simulink model "GalvoModel_v60"  (R2015a)
settings: Solver=ode45  StartTime=0.0  StopTime=5  MaxStep=1e-4  RelTol=1e-3
InitFcn:
  | param=evalin('base','param;');
  | 
  | JR=str2num(param.JR);
  | KMT=str2num(param.KMT);
  | Rc=str2num(param.Rc);
  | Lc=str2num(param.Lc);
  | KFR=str2num(param.KFR);
  | KTB=str2num(param.KTB);
  | KBM=str2num(param.KBM);
  | Rsh=str2num(param.Rsh);
StartFcn:
  | sprintf('Info (%s):\nKTB = %.1e\nKBM = %.1e\n', gcs, KTB, KBM)
model workspace (MATLAB code in the model file):
  | %param=evalin('base','loadGalvoParam(4);');
  | param=evalin('base','param;');
  | 
  | JR=str2num(param.JR);
  | KMT=str2num(param.KMT);
  | Rc=str2num(param.Rc);
  | Lc=str2num(param.Lc);
  | KFR=str2num(param.KFR);
  | KTB=str2num(param.KTB);
  | KBM=str2num(param.KBM);
  | Rsh=str2num(param.Rsh);
undefined symbols (not defined in the file): FS
settings Model: Creator=mainster  LastModifiedBy=mainster
settings DataIOCC: SaveOutput=off  SaveTime=off
settings OptimizationCC: InlineParams=on  BufferReuse=off
settings DebuggingCC: UnderspecifiedInitializationDetection=Classic  MergeDetectMultiDrivingBlocksExec=none  SolverPrmCheckMsg=warning  StateNameClashWarn=warning  InitInArrayFormatMsg=none
settings ModelReferenceCC: ModelReferenceMinAlgLoopOccurrences=on

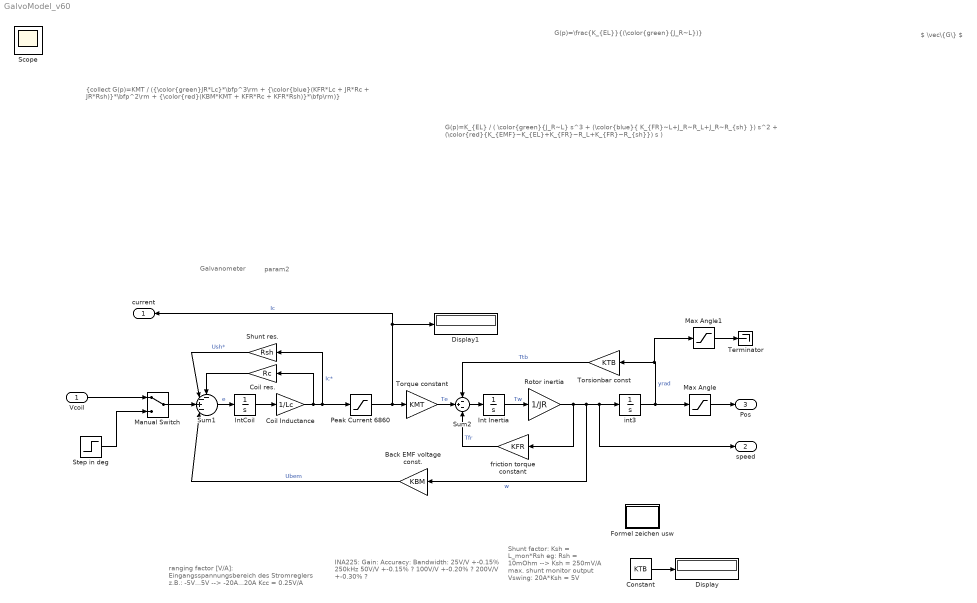
== system GalvoModel_v60 ==
  note: $ \vec\{G\} $
  note: G(p)=\frac{K_{EL}}{(\color{green}{J_R~L})}
  note: G(p)=K_{EL} / ( \color{green}{J_R~L} s^3 + (\color{blue}{ K_{FR}~L+J_R~R_L+J_R~R_{sh} }) s^2 + (\color{red}{K_{EMF}~K_{EL}+K_{FR}~R_L+K_{FR}~R_{sh}}) s )
  note: {collect G(p)=KMT / ({\color{green}JR*Lc}*\bfp^3\rm + {\color{blue}(KFR*Lc + JR*Rc + JR*Rsh)}*\bfp^2\rm + {\color{red}(KBM*KMT + KFR*Rc + KFR*Rsh)}*\bfp\rm)}
  note: param2
  note: Galvanometer
  note: ranging factor [V/A]:
      | Eingangsspannungsbereich des
      | Stromreglers z.B.:
      | -5V...5V --> -20A...20A
      | Kcc = 0.25V/A
  note: Shunt factor:
      | Ksh = L_mon*Rsh
      |
      | eg: Rsh = 10mOhm
      |
      | --> Ksh = 250mV/A
      | max. shunt monitor
      | output Vswing:
      | 20A*Ksh = 5V
  note: INA225:
      | Gain:		Accuracy:		Bandwidth:
      | 25V/V		+-0.15%		250kHz
      | 50V/V		+-0.15%		?
      | 100V/V	+-0.20%		?
      | 200V/V	+-0.30%		?
  Vcoil : Inport
  Back EMF voltage const. : Gain  Gain=KBM
  Coil Inductance : Gain  Gain=1/Lc
  Coil res. : Gain  Gain=Rc
  Constant : Constant  Value=KTB  SampleTime=-1
  Display : Display
  Display1 : Display
  Formel zeichen usw : Subsystem
  Int Inertia : Integrator
  IntCoil : Integrator
  Manual Switch : ManualSwitch
  Max Angle : Saturate  UpperLimit=20*pi/180  LowerLimit=-20*pi/180
      settings: AttributesFormatString=Max=%<UpperLimit>\nMin=%<LowerLimit>
  Max Angle1 : Saturate  UpperLimit=20  LowerLimit=-20
      settings: AttributesFormatString=Max=%<UpperLimit>\nMin=%<LowerLimit>
  Peak Current 6860 : Saturate  UpperLimit=30  LowerLimit=-30
      settings: AttributesFormatString=+-%<UpperLimit>A
  Rotor inertia : Gain  Gain=1/JR
  Shunt res. : Gain  Gain=Rsh
  Step in deg : Step  Time=1e-3  SampleTime=FS  ZeroCross=off
      settings: AttributesFormatString=Ampl.: %<After>\ntime:%<Time>
  Sum1 : Sum  Inputs=--+-|
  Sum2 : Sum  Inputs=-+-
  Terminator : Terminator
  Torque constant : Gain  Gain=KMT
  Torsionbar const : Gain  Gain=KTB
  friction torque constant : Gain  Gain=KFR
  int3 : Integrator
  current : Outport
  speed : Outport  Port=2
  Pos : Outport  Port=3
  Scope : Scope  NumInputPorts=5
      settings: ShowLegends=on  TimeRange=0.015  YMin=0~0~0~-5~-5  YMax=70~0.35~20~5~5  MaxDataPoints=7500
  wires:
  Shunt res./1 -> Sum1/2  "Ush*"
  Coil res./1 -> Sum1/1
  Vcoil/1 -> Manual Switch/1
  Back EMF voltage const./1 -> Sum1/4  "Ubem"
  int3/1 -> Max Angle/1, Max Angle1/1, Torsionbar const/1  "yrad"
  Torque constant/1 -> Sum2/2  "Te"
  Coil Inductance/1 -> Coil res./1, Shunt res./1, Peak Current 6860/1  "Ic*"
  Torsionbar const/1 -> Sum2/1  "Ttb"
  IntCoil/1 -> Coil Inductance/1
  Sum1/1 -> IntCoil/1  "e"
  Int Inertia/1 -> Rotor inertia/1  "Tw"
  Sum2/1 -> Int Inertia/1
  Rotor inertia/1 -> friction torque constant/1, speed/1, int3/1, Back EMF voltage const./1  "w"
  friction torque constant/1 -> Sum2/3  "Tfr"
  Constant/1 -> Display/1
  Max Angle/1 -> Pos/1
  Peak Current 6860/1 -> Display1/1, current/1, Torque constant/1  "Ic"
  Manual Switch/1 -> Sum1/3
  Step in deg/1 -> Manual Switch/2
  Max Angle1/1 -> Terminator/1

== system GalvoModel_v60/Formel zeichen usw ==
  note: Te: 		electrical torque, gen. by coils		[Nm]
      |  Ic: 			coil current							[A]
      |  Tfr:		rotor dynamic friction torque 		[Nm]
      |  Trb:		torsion bar torque					[Nm]
      |  Tw:		angular momentum				[Nm*s]
      |  w:			angular velocity 					[rad/s]
      |  yrad:		angular position 					[rad]
      |  ydeg:		angular position 					[°]
      |  Ucci:		current controller input				[V]
      |  Ucco:		current controller output			[V]
      |  Ush:		shunt voltage						[V]
  note: balance of force: 	Te=Ttb+Tfr
      | 					Te - (Ttb+Tfr)=0  ->  no movement
      |
      |  integrate( 1 Nm )dt = 1 Nm*s
      |  (Nm*s)(kg*m²)⁻¹ = (N*s/kg)*m⁻¹ = m/(s*m) = rad
  note: L_{c  }	coil inductance 							[H]
      |  R_{c  }	coil resistance							[\Omega]
      |  R_{SH }	current shunt resistance				[\Omega]
      |  J_{R  }	rotor inertia 							[kg*m²]
      |  \color{red}K_{TB }	torsion bar torque const. 			[Nm/rad]
      |  \color{black}K_{BM }	back EMF const.							[V*s/rad]
      |  K_{FR }	rotor dyn. friction torque const.	[Nm*s/rad]
      |  K_{MT }	el. magnetic torque const.			[Nm/A]
